simulink model "modify_test1"  (R2013a)
settings: Solver=FixedStepDiscrete  StartTime=0  StopTime=inf  FixedStep=0.001  RelTol=1e-3
PreLoadFcn:
  | RIP_LQR
undefined symbols (not defined in the file): k, K1, K2, K3, K4, Rho
libraries: c280xlib x5, simulink x1
CloseFcn:
  | rtwprivate ssgencode ModelCloseRequest test1
settings Model: Creator=maydinli  LastModifiedBy=vsscloud
settings DataIOCC: SignalLoggingSaveFormat=ModelDataLogs  SaveOutput=off  SaveTime=off  SignalLoggingName=logsOut
settings OptimizationCC: ExpressionDepthLimit=2147483647  InitFltsAndDblsToZero=on  OptimizeModelRefInitCode=on
settings DebuggingCC: SaveWithParameterizedLinksMsg=none  CheckExecutionContextPreStartOutputMsg=on  CheckExecutionContextRuntimeOutputMsg=on  SignalResolutionControl=TryResolveAllWithWarning  MultiTaskDSMMsg=warning  MultiTaskCondExecSysMsg=none  FcnCallInpInsideContextMsg=UseLocalSettings  StrictBusMsg=None
settings HardwareCC: ProdBitPerChar=16  ProdBitPerInt=16  ProdBitPerPointer=16  ProdLargestAtomicInteger=Integer  ProdIntDivRoundTo=Zero  ProdEndianess=LittleEndian  ProdWordSize=16  ProdHWDeviceType=Texas Instruments->C2000  TargetBitPerChar=16  TargetBitPerInt=16  TargetBitPerPointer=16  TargetLargestAtomicInteger=Integer  TargetIntDivRoundTo=Zero  TargetEndianess=LittleEndian  TargetWordSize=16  TargetHWDeviceType=TI C2000
settings RTWCC: SystemTargetFile=idelink_ert.tlc  GenerateMakefile=off  TemplateMakefile=none  Description=Link for CCS (ERT) code generation for TMS320(TM) DSP platforms  ProcessScript=ccslink_ert_make_rtw_hook  IncludeERTFirstTime=on
settings CodeAppCC: IgnoreCustomStorageClasses=off  CustomSymbolStrType=$N$R$M  InternalIdentifier=Classic
settings TargetHardwareResources: Description=Target Hardware Resources Component

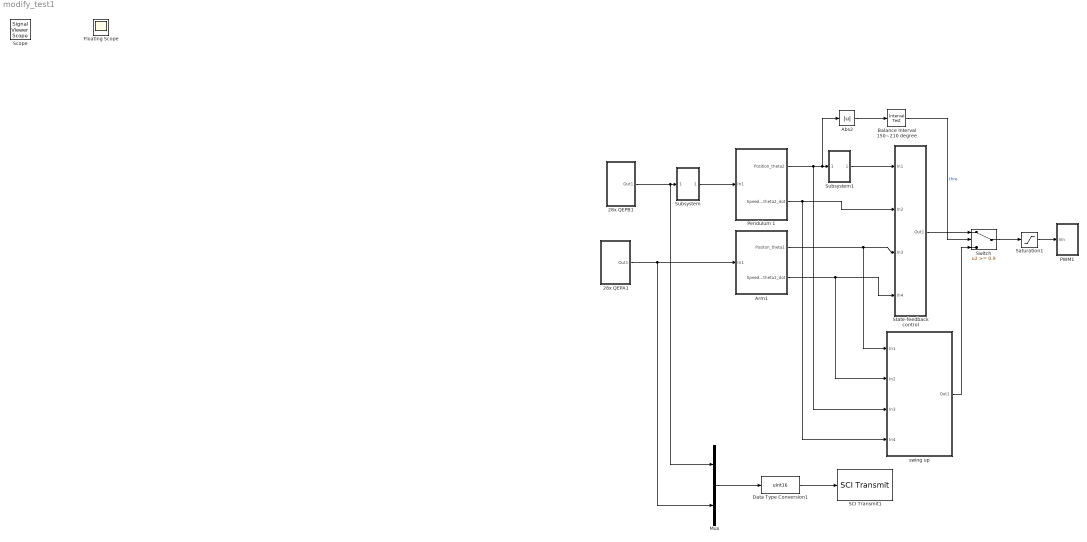
== system modify_test1 ==
  28x QEPA1 : Subsystem
  28x QEPB1 : Subsystem
  Abs2 : Abs  SaturateOnIntegerOverflow=on
  Arm1 : Subsystem
  Balance Interval 150~210 degree : simulink/Logic and Bit Operations/Interval Test  IntervalClosedRight=on  uplimit=2*pi/360*195  IntervalClosedLeft=on  lowlimit=2*pi/360*165  OutDataTypeStr=boolean
  Data Type Conversion1 : DataTypeConversion  OutDataTypeStr=uint16  SampleTime=0.001
  Mux : Mux  Inputs=2
  PWM1 : Subsystem
  Pendulum 1 : Subsystem
  SCI Transmit1 : c280xlib/SCI Transmit  sciModule=A  dataHead=222  dataTail=253  postInterrupt=on  numFifo=0
  Saturation1 : Saturate  UpperLimit=12  LowerLimit=-12
  State-feedback control : Subsystem
  Subsystem : Subsystem
  Subsystem1 : Subsystem
  Switch : Switch  Threshold=0.9
  "swing up " : Subsystem
  Floating Scope : Scope
      settings: Floating=on
  Scope : SignalViewerScope  IOType=viewer  RefreshTime=0.035000
  wires:
  Data Type Conversion1/1 -> SCI Transmit1/1
  Mux/1 -> Data Type Conversion1/1
  28x QEPA1/1(Out1) -> Mux/2, Arm1/1(In1)
  Saturation1/1 -> PWM1/1(Vin)
  Arm1/1(Positon_theta1) -> "swing up "/1(In1), State-feedback control/3(In3)
  Arm1/2(Speed_theta1_dot) -> "swing up "/2(In2), State-feedback control/4(In4)
  28x QEPB1/1(Out1) -> Mux/1, Subsystem/1(In1)
  Subsystem/1(Out1) -> Pendulum 1/1(In1)
  Switch/1 -> Saturation1/1
  State-feedback control/1(Out1) -> Switch/1
  Subsystem1/1(Out1) -> State-feedback control/1(In1)
  Abs2/1 -> Balance Interval 150~210 degree/1
  Balance Interval 150~210 degree/1 -> Switch/2  "thre"
  "swing up "/1(Out1) -> Switch/3
  Pendulum 1/1(Position_theta2) -> "swing up "/3(In3), Abs2/1, Subsystem1/1(In1)
  Pendulum 1/2(Speed_theta2_dot) -> "swing up "/4(In4), State-feedback control/2(In2)

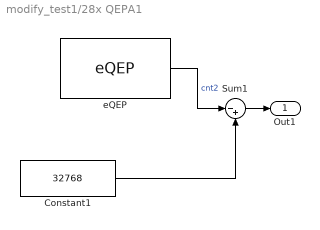
== system modify_test1/28x QEPA1 ==
  Constant1 : Constant  Value=32768
  Sum1 : Sum  Inputs=|-+
  eQEP : c280xlib/eQEP  useModule=eQEP2  pcInputmode=Quadrature-count  externalClockrate=2x resolution: Count the rising/falling edge  swapPolarityselection=Clockwise  qdfOutputport=off  qapPolarityselection=off  qbpPolarityselection=off  qipPolarityselection=off  qspPolarityselection=off  igatePolarityselection=off  sampleTime=0.001  pcOutputport=on  pcMaximumvalue=4294967295  indexInitializationcheck=off  indexInitializationevent=Rising edge  strobeInitializationcheck=off  strobeInitializationevent=Rising edge  softwareInitializationcheck=on  softwareInitializationsource=Set to init value at start up  softwareInitializationmode=on  pcInitialvalue=32768  pcResetmode=Reset on an index event  ieloutputport=off  indexEventlatch=Rising edge  seloutputport=off  strobeEventlatch=Rising edge  pcefOutputport=off  enableEqepcapture=off  qctmrOutputport=off  qcprdOutputport=off  captureTimerprescaler=128  upEventprescaler=128  overflowErrorflag=off  directionErrorflag=off  captureTimerposition=On position counter read  unitTimerperiod=100000000  captureTimerlatch=off  capturePeriodlatch=off  positionCounterlatch=off  soenPolarityselection=off  spselPolarityselection=Index pin is used for sync output  compareValuesource=Specify via dialog  shadowMode=Load on QPOSCNT=0  compareValue=4294967295  syncOutputwidth=1  polaritySyncoutput=Active high  watchdogEnable=off  watchdogTimer=65535  outport1Datatype=auto  outport2Datatype=auto  outport3Datatype=auto  outport4Datatype=auto  outport5Datatype=auto  outport6Datatype=auto  outport7Datatype=auto  outport8Datatype=auto  outport9Datatype=auto  outport10Datatype=auto  outport11Datatype=auto  outport12Datatype=auto  eqepinterrupt_pce=off  eqepinterrupt_qpe=off  eqepinterrupt_qdc=off  eqepinterrupt_wto=off  eqepinterrupt_pcu=off  eqepinterrupt_pco=off  eqepinterrupt_pcr=off  eqepinterrupt_pcm=off  eqepinterrupt_sel=off  eqepinterrupt_iel=off  eqepinterrupt_uto=off  pheOutputport=off  watchdogOutputport=off  outport13Datatype=auto  outport14Datatype=auto
  Out1 : Outport
  wires:
  Sum1/1 -> Out1/1
  Constant1/1 -> Sum1/2
  eQEP/1 -> Sum1/1  "cnt2"

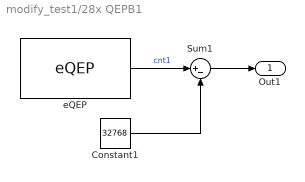
== system modify_test1/28x QEPB1 ==
  Constant1 : Constant  Value=32768
  Sum1 : Sum  Inputs=|+-
  eQEP : c280xlib/eQEP  useModule=eQEP1  pcInputmode=Quadrature-count  externalClockrate=2x resolution: Count the rising/falling edge  swapPolarityselection=Clockwise  qdfOutputport=off  qapPolarityselection=off  qbpPolarityselection=off  qipPolarityselection=off  qspPolarityselection=off  igatePolarityselection=off  sampleTime=0.001  pcOutputport=on  pcMaximumvalue=4294967295  indexInitializationcheck=off  indexInitializationevent=Rising edge  strobeInitializationcheck=off  strobeInitializationevent=Rising edge  softwareInitializationcheck=on  softwareInitializationsource=Set to init value at start up  softwareInitializationmode=on  pcInitialvalue=32768  pcResetmode=Reset on an index event  ieloutputport=off  indexEventlatch=Rising edge  seloutputport=off  strobeEventlatch=Rising edge  pcefOutputport=off  enableEqepcapture=off  qctmrOutputport=off  qcprdOutputport=off  captureTimerprescaler=128  upEventprescaler=128  overflowErrorflag=off  directionErrorflag=off  captureTimerposition=On position counter read  unitTimerperiod=100000000  captureTimerlatch=off  capturePeriodlatch=off  positionCounterlatch=off  soenPolarityselection=off  spselPolarityselection=Index pin is used for sync output  compareValuesource=Specify via dialog  shadowMode=Load on QPOSCNT=0  compareValue=4294967295  syncOutputwidth=1  polaritySyncoutput=Active high  watchdogEnable=off  watchdogTimer=65535  outport1Datatype=auto  outport2Datatype=auto  outport3Datatype=auto  outport4Datatype=auto  outport5Datatype=auto  outport6Datatype=auto  outport7Datatype=auto  outport8Datatype=auto  outport9Datatype=auto  outport10Datatype=auto  outport11Datatype=auto  outport12Datatype=auto  eqepinterrupt_pce=off  eqepinterrupt_qpe=off  eqepinterrupt_qdc=off  eqepinterrupt_wto=off  eqepinterrupt_pcu=off  eqepinterrupt_pco=off  eqepinterrupt_pcr=off  eqepinterrupt_pcm=off  eqepinterrupt_sel=off  eqepinterrupt_iel=off  eqepinterrupt_uto=off  pheOutputport=off  watchdogOutputport=off  outport13Datatype=auto  outport14Datatype=auto
  Out1 : Outport
  wires:
  Constant1/1 -> Sum1/2
  eQEP/1 -> Sum1/1  "cnt1"
  Sum1/1 -> Out1/1

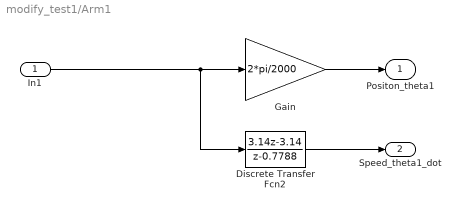
== system modify_test1/Arm1 ==
  In1 : Inport
  Discrete Transfer Fcn2 : DiscreteTransferFcn  Numerator=[3.14 -3.14]  Denominator=[1 -0.7788]  SampleTime=0.001
  Gain : Gain  Gain=2*pi/2000  SaturateOnIntegerOverflow=on  OutDataTypeStr=Inherit: Same as input  ParamDataTypeStr=Inherit: Same as input
  Positon_theta1 : Outport
  Speed_theta1_dot : Outport  Port=2
  wires:
  In1/1 -> Gain/1, Discrete Transfer Fcn2/1
  Discrete Transfer Fcn2/1 -> Speed_theta1_dot/1
  Gain/1 -> Positon_theta1/1

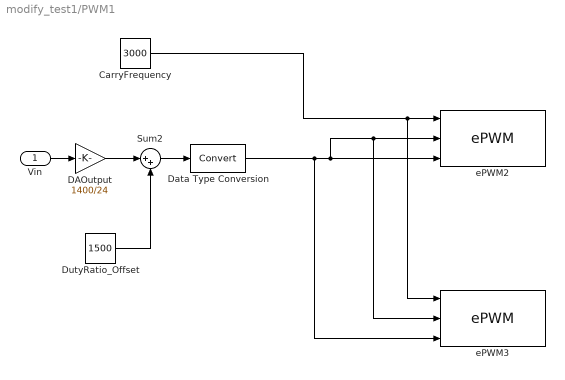
== system modify_test1/PWM1 ==
  Vin : Inport
  CarryFrequency : Constant  Value=3000  OutDataTypeStr=uint16
  DAOutput : Gain  Gain=1400/24  SaturateOnIntegerOverflow=on  OutDataTypeStr=Inherit: Same as input  ParamDataTypeStr=Inherit: Same as input
  Data Type Conversion : DataTypeConversion  SaturateOnIntegerOverflow=on  RndMeth=Zero
  DutyRatio_Offset : Constant  Value=1500
  Sum2 : Sum  Inputs=|++  SaturateOnIntegerOverflow=on
  ePWM2 : c280xlib/ePWM  checkMode=off  useModule=ePWM1  periodUnits=Clock cycles  timerSource=Input port  timerPeriod_clk=3000  timerPeriod_sec=0.0001  tbshadow=Counter equals to zero  countingMode=Up  phaseActiveEnable=Disable  phaseDirection=Count down after sync  phaseActive=0  synchronizationEnable=off  synchronizationOption=Disable  clockPrescale=1  HSclockPrescale=1  ePWMxAStatus=on  CMPAUnits=Clock cycles  CMPASource=Input port  CMPAValue_per=50  CMPAValue_clk=1500  enCMPAshadow=Counter equals to zero  ePWMxAactionLogic1=Do nothing  ePWMxAactionLogic2=Clear  ePWMxAactionLogic3=Set  ePWMxAactionLogic4=Do nothing  ePWMxAactionLogic5=Do nothing  ePWMxAactionLogic6=Do nothing  ePWMxALoadMode=Load on counter equals to zero (CTR=Zero)  ePWMxACSFenable=off  ePWMxACSFvalue=Forcing disable  ePWMxASFreload=Zero  enHRPWM=off  HRPWM_LoadMode=Counter equals to zero (CTR=ZERO)  HRPWM_CTLMode=Phase control mode  HRPWM_EDGMode=Both edge  enSFO=on  ePWMxBStatus=on  CMPBUnits=Clock cycles  CMPBSource=Input port  CMPBValue_per=50  CMPBValue_clk=1500  enCMPBshadow=Counter equals to zero  ePWMxBactionLogic1=Do nothing  ePWMxBactionLogic2=Set  ePWMxBactionLogic3=Do nothing  ePWMxBactionLogic4=Do nothing  ePWMxBactionLogic5=Clear  ePWMxBactionLogic6=Do nothing  ePWMxBLoadMode=Load on counter equals to zero (CTR=Zero)  ePWMxBCSFenable=off  ePWMxBCSFvalue=Forcing disable  ePWMxBSFreload=Zero  enableDBePWMxA=on  enableDBePWMxB=on  DBpolarity=Active high complementary (AHC)  DBedgeDelay=Positive  DBSource_ePWMxA=ePWMxA  DBSource_ePWMxB=ePWMxA  DBperiodSource=Specify via dialog  REDperiod=102  FEDperiod=102  adcstartModuleA=off  adcrequestEventA=First event  adcstartEventA=Counter equals to zero (CTR=Zero)  adcstartModuleB=off  adcrequestEventB=First event  adcstartEventB=Counter equals to zero (CTR=Zero)  intEn=off  intPrd=First event  intSel=Counter equals to zero (CTR=Zero)  chopperEnable=off  chopperFrequency=1  chopperFirstwidth=1  chopperDuty=12.5%  tripZonesource=Specify via dialog  tzselOSHT1=off  tzselOSHT2=off  tzselOSHT3=off  tzselOSHT4=off  tzselOSHT5=off  tzselOSHT6=off  tzselCBC1=off  tzselCBC2=off  tzselCBC3=off  tzselCBC4=off  tzselCBC5=off  tzselCBC6=off  enTzOstIntr=off  enTzCbcIntr=off  ePWMxAforced=No action  ePWMxBforced=No action  timerPeriod=-1  ePWMxAValue=0  ePWMxBValue=0  tripZoneoption=One-shot trip (OSHT)
  ePWM3 : c280xlib/ePWM  checkMode=off  useModule=ePWM2  periodUnits=Clock cycles  timerSource=Input port  timerPeriod_clk=3000  timerPeriod_sec=0.0001  tbshadow=Counter equals to zero  countingMode=Up  phaseActiveEnable=Disable  phaseDirection=Count down after sync  phaseActive=0  synchronizationEnable=off  synchronizationOption=Disable  clockPrescale=1  HSclockPrescale=1  ePWMxAStatus=on  CMPAUnits=Clock cycles  CMPASource=Input port  CMPAValue_per=50  CMPAValue_clk=1500  enCMPAshadow=Counter equals to zero  ePWMxAactionLogic1=Do nothing  ePWMxAactionLogic2=Clear  ePWMxAactionLogic3=Set  ePWMxAactionLogic4=Do nothing  ePWMxAactionLogic5=Do nothing  ePWMxAactionLogic6=Do nothing  ePWMxALoadMode=Load on counter equals to zero (CTR=Zero)  ePWMxACSFenable=off  ePWMxACSFvalue=Forcing disable  ePWMxASFreload=Zero  enHRPWM=off  HRPWM_LoadMode=Counter equals to zero (CTR=ZERO)  HRPWM_CTLMode=Phase control mode  HRPWM_EDGMode=Both edge  enSFO=on  ePWMxBStatus=on  CMPBUnits=Clock cycles  CMPBSource=Input port  CMPBValue_per=50  CMPBValue_clk=1500  enCMPBshadow=Counter equals to zero  ePWMxBactionLogic1=Do nothing  ePWMxBactionLogic2=Set  ePWMxBactionLogic3=Do nothing  ePWMxBactionLogic4=Do nothing  ePWMxBactionLogic5=Clear  ePWMxBactionLogic6=Do nothing  ePWMxBLoadMode=Load on counter equals to zero (CTR=Zero)  ePWMxBCSFenable=off  ePWMxBCSFvalue=Forcing disable  ePWMxBSFreload=Zero  enableDBePWMxA=on  enableDBePWMxB=on  DBpolarity=Active high complementary (AHC)  DBedgeDelay=Positive  DBSource_ePWMxA=ePWMxA  DBSource_ePWMxB=ePWMxA  DBperiodSource=Specify via dialog  REDperiod=204  FEDperiod=204  adcstartModuleA=off  adcrequestEventA=First event  adcstartEventA=Counter equals to zero (CTR=Zero)  adcstartModuleB=off  adcrequestEventB=First event  adcstartEventB=Counter equals to zero (CTR=Zero)  intEn=off  intPrd=First event  intSel=Counter equals to zero (CTR=Zero)  chopperEnable=off  chopperFrequency=1  chopperFirstwidth=1  chopperDuty=12.5%  tripZonesource=Specify via dialog  tzselOSHT1=off  tzselOSHT2=off  tzselOSHT3=off  tzselOSHT4=off  tzselOSHT5=off  tzselOSHT6=off  tzselCBC1=off  tzselCBC2=off  tzselCBC3=off  tzselCBC4=off  tzselCBC5=off  tzselCBC6=off  enTzOstIntr=off  enTzCbcIntr=off  ePWMxAforced=No action  ePWMxBforced=No action  timerPeriod=-1  ePWMxAValue=0  ePWMxBValue=0  tripZoneoption=One-shot trip (OSHT)
  wires:
  DAOutput/1 -> Sum2/1
  Vin/1 -> DAOutput/1
  Data Type Conversion/1 -> ePWM2/2, ePWM3/2, ePWM2/3, ePWM3/3
  Sum2/1 -> Data Type Conversion/1
  CarryFrequency/1 -> ePWM2/1, ePWM3/1
  DutyRatio_Offset/1 -> Sum2/2

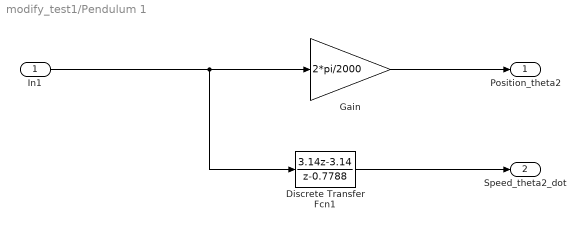
== system modify_test1/Pendulum 1 ==
  In1 : Inport
  Discrete Transfer Fcn1 : DiscreteTransferFcn  Numerator=[3.14 -3.14]  Denominator=[1 -0.7788]  SampleTime=0.001
  Gain : Gain  Gain=2*pi/2000  SaturateOnIntegerOverflow=on  OutDataTypeStr=Inherit: Same as input  ParamDataTypeStr=Inherit: Same as input
  Position_theta2 : Outport
  Speed_theta2_dot : Outport  Port=2
  wires:
  In1/1 -> Gain/1, Discrete Transfer Fcn1/1
  Discrete Transfer Fcn1/1 -> Speed_theta2_dot/1
  Gain/1 -> Position_theta2/1

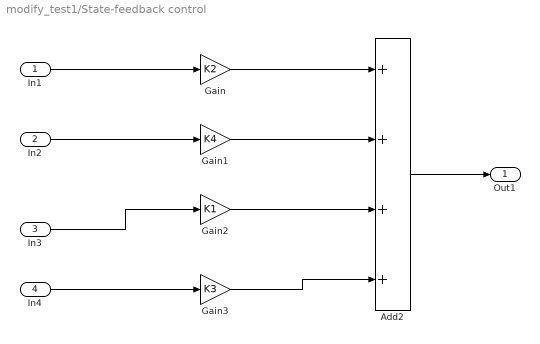
== system modify_test1/State-feedback control ==
  In1 : Inport
  In2 : Inport  Port=2
  In3 : Inport  Port=3
  In4 : Inport  Port=4
  Add2 : Sum  Inputs=++++
  Gain : Gain  Gain=K2
  Gain1 : Gain  Gain=K4
  Gain2 : Gain  Gain=K1
  Gain3 : Gain  Gain=K3
  Out1 : Outport
  wires:
  Gain2/1 -> Add2/3
  In1/1 -> Gain/1
  Gain/1 -> Add2/1
  Gain1/1 -> Add2/2
  Add2/1 -> Out1/1
  In4/1 -> Gain3/1
  In2/1 -> Gain1/1
  In3/1 -> Gain2/1
  Gain3/1 -> Add2/4

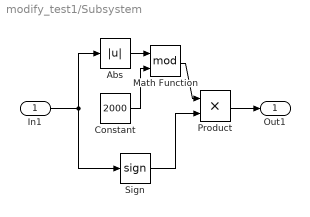
== system modify_test1/Subsystem ==
  In1 : Inport
  Abs : Abs
  Constant : Constant  Value=2000
  Math Function : Math  Operator=mod  SaturateOnIntegerOverflow=on
  Product : Product
  Sign : Signum
  Out1 : Outport
  wires:
  Constant/1 -> Math Function/2
  Abs/1 -> Math Function/1
  Sign/1 -> Product/2
  Product/1 -> Out1/1
  Math Function/1 -> Product/1
  In1/1 -> Sign/1, Abs/1

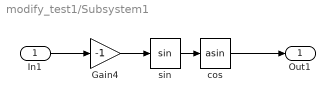
== system modify_test1/Subsystem1 ==
  In1 : Inport
  Gain4 : Gain  Gain=-1  SaturateOnIntegerOverflow=on  OutDataTypeStr=Inherit: Same as input  ParamDataTypeStr=Inherit: Same as input
  cos : Trigonometry  Operator=asin
  sin : Trigonometry
  Out1 : Outport
  wires:
  cos/1 -> Out1/1
  In1/1 -> Gain4/1
  sin/1 -> cos/1
  Gain4/1 -> sin/1

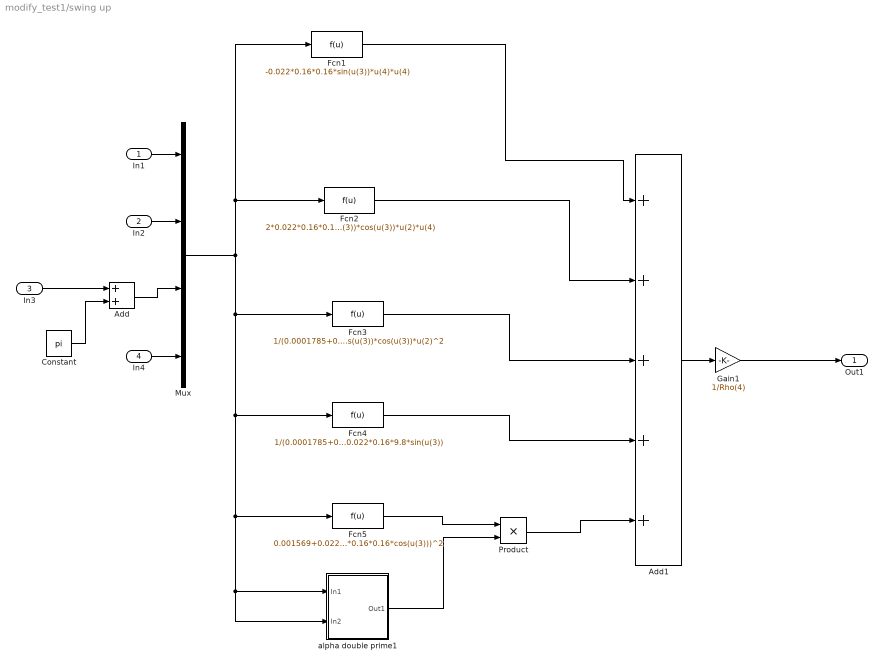
== system modify_test1/swing up  ==
  In1 : Inport
  In2 : Inport  Port=2
  In3 : Inport  Port=3
  In4 : Inport  Port=4
  Add : Sum
  Add1 : Sum  Inputs=+++++
  Constant : Constant  Value=pi
  Fcn1 : Fcn  Expr=-0.022*0.16*0.16*sin(u(3))*u(4)*u(4)
  Fcn2 : Fcn  Expr=2*0.022*0.16*0.16*sin(u(3))*cos(u(3))*u(2)*u(4)
  Fcn3 : Fcn  Expr=1/(0.0001785+0.022*0.16*0.16)*0.022^2*0.16^4*sin(u(3))*cos(u(3))*cos(u(3))*u(2)^2
  Fcn4 : Fcn  Expr=1/(0.0001785+0.022*0.16*0.16)*0.022*0.16*0.16*cos(u(3))*0.022*0.16*9.8*sin(u(3))
  Fcn5 : Fcn  Expr=0.001569+0.022*(0.16*0.16+0.16*0.16*(sin(u(3)))^2)-1/(0.0001785+0.022*0.16*0.16)*(0.022*0.16*0.16*cos(u(3)))^2
  Gain1 : Gain  Gain=1/Rho(4)
  Mux : Mux
  Product : Product
  alpha double prime1 : Subsystem
  Out1 : Outport
  wires:
  In4/1 -> Mux/4
  In2/1 -> Mux/2
  In1/1 -> Mux/1
  Gain1/1 -> Out1/1
  Mux/1 -> Fcn2/1, Fcn1/1, alpha double prime1/2(In2), alpha double prime1/1(In1), Fcn5/1, Fcn4/1, Fcn3/1
  Constant/1 -> Add/2
  In3/1 -> Add/1
  Add/1 -> Mux/3
  Fcn5/1 -> Product/1
  alpha double prime1/1(Out1) -> Product/2
  Fcn1/1 -> Add1/1
  Fcn2/1 -> Add1/2
  Fcn3/1 -> Add1/3
  Fcn4/1 -> Add1/4
  Product/1 -> Add1/5
  Add1/1 -> Gain1/1

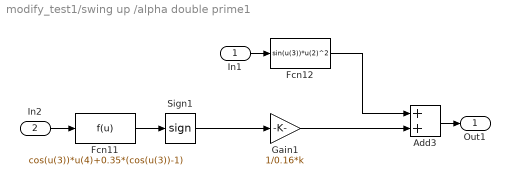
== system modify_test1/swing up /alpha double prime1 ==
  In1 : Inport
  In2 : Inport  Port=2
  Add3 : Sum
  Fcn11 : Fcn  Expr=cos(u(3))*u(4)+0.35*(cos(u(3))-1)
  Fcn12 : Fcn  Expr=sin(u(3))*u(2)^2
  Gain1 : Gain  Gain=1/0.16*k
  Sign1 : Signum
  Out1 : Outport
  wires:
  In2/1 -> Fcn11/1
  Add3/1 -> Out1/1
  In1/1 -> Fcn12/1
  Fcn12/1 -> Add3/1
  Gain1/1 -> Add3/2
  Fcn11/1 -> Sign1/1
  Sign1/1 -> Gain1/1
